simulink model "BEML_EMU"  (R2019b)
settings: configuration reference "ConfigSet_SimIntegration" (kept outside this file)
model workspace (MAT data in the model file):
  BrakesSampleTime = 0.01
  ConfigSampleTime = 0.05
  CouplingSampleTime = 0.05
  DoorsSampleTime = 0.05
  DynamicsSampleTime = 0.001
  ElectricalSampleTime = 0.05
  PRM_SimIntegration : Simulink.Parameter (value not decoded)
  PantographSampleTime = 0.05
  PneumaticsSampleTime = 0.01
  SampleTime = 0.001
  TractionSampleTime = 0.01
undefined symbols (not defined in the file): Acceleration, AngularAcceleration, AngularVelocity, BrakeFadeEnable, Brakes, BrakeShoeCoefficientCalculationMethod, BrakeShoeFrictionCoeff, BrakeTemperatureEnable, Common, DampingAdjustmentDesignMass, DavisCoeffA1, DavisCoeffA2, DavisCoeffB1, DavisCoeffB2, DavisCoefficients, DavisCoeffLeadCarC, DavisCoeffTailCarC, DiscIntNeverNeededParam, Doors, DragCalculationMethod, Dynamics, Effects, Electrical, EnableDampingAdjustmentByMass, Environment, Equipment, ExternalEffects, H, HasMotor, HasPanto, HornActivation, IsFirstVehicle, IsLastVehicle, isLeft, IsNonCab, LateralJolt, Location, LongitudinalJolt, MaxVehicles, MotionBaseSafetyCutout, OrientationDCM, P, Pantograph, Pneumatics, PneumaticsPoweredPanto, R, Traction, Transform, Tuning, UnitConfig, Velocity, VerticalJolt, VerticalJoltDown, VigilanceIntervention
libraries: simulink x35, IOStateMachinesLib x26, TestBenchLib x6, LatchesLib x3, BEML_EMU_BrakesInput_Lib x1, BEML_EMU_CBTCInterface_Lib x1, BEML_EMU_Couplers_Lib x1, BEML_EMU_DoorsInput_Lib x1, BEML_EMU_DynamicsInput_Lib x1, BEML_EMU_ElectricalInput_Lib x1, BEML_EMU_PantographInput_Lib x1, BEML_EMU_PneumaticsInput_Lib x1
(part 5 of 6)

== system BEML_EMU/InputsInterface/VehicleConfigProcessing/VehicleConfigInterface/VehicleConfigInterface/AssignTraction ==
  In Bus Element : Inport  PortName=VehicleConfig  Element=Common.Class
  Data Type Conversion : DataTypeConversion
  Merge1 : Merge  Inputs=4
  Switch Case2 : SwitchCase  CaseConditions={[101], [102], [103]}
  VehicleEquipment : Subsystem  mask(Tram Vehicle Equipment){HasMotors=on}
      mask prompts: HasMotors "Has Motors?"
      mask DialogControl ParameterGroupVar Prompt: Equipment
  VehicleEquipment1 : Subsystem  mask(Tram Vehicle Equipment){HasMotors=off}
      mask prompts: HasMotors "Has Motors?"
      mask DialogControl ParameterGroupVar Prompt: Equipment
  VehicleEquipment2 : Subsystem  mask(Tram Vehicle Equipment){HasMotors=on}
      mask prompts: HasMotors "Has Motors?"
      mask DialogControl ParameterGroupVar Prompt: Equipment
  VehicleEquipment3 : Subsystem  mask(Tram Vehicle Equipment){HasMotors=off}
      mask prompts: HasMotors "Has Motors?"
      mask DialogControl ParameterGroupVar Prompt: Equipment
  TractionBus : Outport  VectorParamsAs1DForOutWhenUnconnected=off
  wires:
  VehicleEquipment/1(EquipmentBus) -> Merge1/1
  Switch Case2/2 -> VehicleEquipment1/Action
  Merge1/1 -> TractionBus/1
  Switch Case2/4 -> VehicleEquipment3/Action
  Data Type Conversion/1 -> Switch Case2/1  "VehicleClasEnum"
  Switch Case2/3 -> VehicleEquipment2/Action
  In Bus Element/1 -> Data Type Conversion/1
  Switch Case2/1 -> VehicleEquipment/Action
  VehicleEquipment3/1(EquipmentBus) -> Merge1/4
  VehicleEquipment1/1(EquipmentBus) -> Merge1/2
  VehicleEquipment2/1(EquipmentBus) -> Merge1/3

== system BEML_EMU/InputsInterface/VehicleConfigProcessing/VehicleConfigInterface/VehicleConfigInterface/Common ==
  Input : Inport
  Bus Assignment3 : BusAssignment  AssignedSignals=NumberOfAxles
  Constant1 : Constant  Value=4  OutDataTypeStr=Inherit: Inherit via back propagation
  Data Type Conversion3 : DataTypeConversion
  Common : Outport  VectorParamsAs1DForOutWhenUnconnected=off
  wires:
  Constant1/1 -> Data Type Conversion3/1
  Data Type Conversion3/1 -> Bus Assignment3/2
  Bus Assignment3/1 -> Common/1
  Input/1 -> Bus Assignment3/1

== system BEML_EMU/InputsInterface/VehicleConfigProcessing/VehicleConfigInterface/VehicleConfigInterface/Dynamics ==
  note: Davis coefficients reused from BJSNA
      |
      | Davis Equation
      | F (N) = A1*Mass + A2 + B1*Mass*Vel + B2*Vel + C*Vel^2
  Dynamics : Inport
  TrainInput : Inport  Port=2
  Bus Assignment : BusAssignment  AssignedSignals=InitialVelocity
  Bus Assignment1 : BusAssignment  AssignedSignals=DragCalculationMethod,EnableDampingAdjustmentByMass,DampingAdjustmentDesignMass,DavisCoefficients
  Bus Assignment2 : BusAssignment  AssignedSignals=DavisCoeffA1,DavisCoeffA2,DavisCoeffB1,DavisCoeffB2,DavisCoeffLeadCarC,DavisCoeffTailCarC
  Bus Selector1 : BusSelector  OutputSignals=Overrides.InitialVelocity
  Constant : Constant  Value=0  OutDataTypeStr=Bus: BD_TrainDynamics_Cfg_Vehicle_DavisCoefficients
  Constant1 : Constant  Value=12.38
  Constant12 : Constant  Value=20e3
  Constant2 : Constant  Value=0
  Constant5 : Constant  Value=0.044e-3
  Constant6 : Constant  Value=5.18*0.8
  Constant7 : Constant  Value=5.18*0.2/7
  Constant8 : Constant  OutDataTypeStr=boolean
  Constant9 : Constant  Value=8.34e-3
  UseDavisCoeff : Constant  Value=DragCalculationMethod.Davis
  DynamicsProcessed : Outport  VectorParamsAs1DForOutWhenUnconnected=off
  wires:
  Dynamics/1 -> Bus Assignment/1
  Bus Selector1/1 -> Bus Assignment/2  "<InitialVelocity>"
  TrainInput/1 -> Bus Selector1/1
  Bus Assignment2/1 -> Bus Assignment1/5
  Constant/1 -> Bus Assignment2/1
  Constant1/1 -> Bus Assignment2/5
  UseDavisCoeff/1 -> Bus Assignment1/2
  Constant9/1 -> Bus Assignment2/2
  Constant2/1 -> Bus Assignment2/3
  Constant5/1 -> Bus Assignment2/4
  Constant7/1 -> Bus Assignment2/7
  Constant8/1 -> Bus Assignment1/3
  Constant6/1 -> Bus Assignment2/6
  Constant12/1 -> Bus Assignment1/4
  Bus Assignment1/1 -> DynamicsProcessed/1
  Bus Assignment/1 -> Bus Assignment1/1

== system BEML_EMU/InputsInterface/VehicleConfigProcessing/VehicleConfigInterface/VehicleConfigInterface/LocationConfig ==
  VehicleEnabled : Inport
  VehicleEnabledUp : Inport  Port=2
  VehicleEnabledDown : Inport  Port=3
  ClassDown : Inport  Port=4
  ClassUp : Inport  Port=5
  UnitID : Inport  Port=6
  In Bus Element1 : Inport  Port=7  PortName=VehicleConfig  Element=Common
  MaxUnit : Inport  Port=8
  AND2 : Logic  AllPortsSameDT=off  OutDataTypeStr=boolean
  AND3 : Logic  AllPortsSameDT=off  OutDataTypeStr=boolean
  Bus Assignment : BusAssignment  AssignedSignals=IsFirstVehicle,IsLastVehicle
  Bus Assignment1 : BusAssignment  AssignedSignals=UnitConfig.UnitID,UnitConfig.UnitConnection
  Constant1 : Constant  Value=0  OutDataTypeStr=Bus: BD_SimIntegration_Cfg_Vehicle_Location
  NOT : Logic  Operator=NOT  AllPortsSameDT=off  OutDataTypeStr=boolean
  NOT1 : Logic  Operator=NOT  AllPortsSameDT=off  OutDataTypeStr=boolean
  Subsystem : Subsystem
  UnitConf : Subsystem
  LocationConfig : Outport  VectorParamsAs1DForOutWhenUnconnected=off
  Enabled : Outport  Port=2
  UnitConnection : Outport  Port=3
  wires:
  Bus Assignment/1 -> Bus Assignment1/1
  AND2/1 -> Bus Assignment/2  "IsFirstVehicle"
  AND3/1 -> Bus Assignment/3  "IsLastVehicle"
  VehicleEnabledDown/1 -> NOT1/1
  NOT/1 -> AND2/2
  VehicleEnabled/1 -> AND3/1, AND2/1
  Constant1/1 -> Bus Assignment/1
  VehicleEnabledUp/1 -> NOT/1
  NOT1/1 -> AND3/2
  UnitConf/1(UnitConnection) -> Bus Assignment1/3, UnitConnection/1  "UnitConnection"
  In Bus Element1/1 -> UnitConf/1(VehicleConfig)
  ClassDown/1 -> UnitConf/2(ClassDown)
  UnitConf/2(Enabled) -> Enabled/1
  ClassUp/1 -> UnitConf/3(ClassUp)
  Bus Assignment1/1 -> LocationConfig/1
  UnitID/1 -> Subsystem/1(UnitID)
  MaxUnit/1 -> Subsystem/2(MaxUnit)
  Subsystem/1(Out2) -> Bus Assignment1/2

== system BEML_EMU/InputsInterface/VehicleConfigProcessing/VehicleConfigInterface/VehicleEnabled/Subsystem ==
  VehicleConfig : Inport  Partition=on  PartitionDimension=1  PartitionWidth=1  PartitionOffset=0
  Bus Selector : BusSelector  OutputSignals=Common.Enabled
  For Each : ForEach  DisableCoverage=on
  Enabled : Outport  ConcatenationDimension=1  VectorParamsAs1DForOutWhenUnconnected=off
  wires:
  VehicleConfig/1 -> Bus Selector/1
  Bus Selector/1 -> Enabled/1  "<Enabled>"

== system BEML_EMU/InputsInterface/VehicleConfigProcessing/VehicleConfigInterface/VehicleEnabled/Subsystem1 ==
  VehicleConfig : Inport  Partition=on  PartitionDimension=1  PartitionWidth=1  PartitionOffset=0
  Bus Selector : BusSelector  OutputSignals=Common.Class
  For Each : ForEach  DisableCoverage=on
  Class : Outport  ConcatenationDimension=1  VectorParamsAs1DForOutWhenUnconnected=off
  wires:
  Bus Selector/1 -> Class/1  "<Class>"
  VehicleConfig/1 -> Bus Selector/1

== system BEML_EMU/SimulatorSystems/ScoringSystemInterface/TrainLevelScoring/For Each Subsystem/Subsystem ==
  <Bogie> : Inport
  Bus Selector1 : BusSelector  OutputSignals=Bogie
  Subsystem : Subsystem
  Out1 : Outport
  Out2 : Outport  Port=2
  wires:
  <Bogie>/1 -> Bus Selector1/1
  Bus Selector1/1 -> Subsystem/1(<Bogie>)  "<Bogie>"
  Subsystem/1(Out1) -> Out1/1
  Subsystem/2(Out2) -> Out2/1

== system BEML_EMU/SimulatorSystems/Subsystem/Input Adapter/MotionBaseInputAdapter/Effects In Processing ==
  note: external effects is "degraded track" and Rough track
  In Bus Element : Inport  PortName=MotionBaseInput  Element=Effects
  Bus Assignment4 : BusAssignment  AssignedSignals=ExternalEffects,LongitudinalJolt,LateralJolt,VerticalJolt,VerticalJoltDown
  Constant : Constant  Value=0  OutDataTypeStr=Bus: BD_MotionBase_In_Vehicle_Effects
  FIXME : TestBenchLib/FIXME
      settings: SourceProductName=Sydac Utilities
  Effects : Outport
  wires:
  Bus Assignment4/1 -> Effects/1  "Effects"
  Constant/1 -> Bus Assignment4/1
  In Bus Element/1 -> Bus Assignment4/2  "Effects"
  FIXME/1 -> Bus Assignment4/6, Bus Assignment4/5, Bus Assignment4/4, Bus Assignment4/3

== system BEML_EMU/SimulatorSystems/Subsystem/Input Adapter/MotionBaseInputAdapter/Environment Dynamics In Processing ==
  Bus Assignment4 : BusAssignment  AssignedSignals=Contact
  Constant10 : Constant  Value=0  OutDataTypeStr=Bus: BD_MotionBase_In_Vehicle_Environment
  Constant5 : Constant  Value=0
  Environment : Outport
  wires:
  Constant10/1 -> Bus Assignment4/1
  Constant5/1 -> Bus Assignment4/2  "Contact"
  Bus Assignment4/1 -> Environment/1  "Environment"

== system BEML_EMU/SimulatorSystems/Subsystem/Input Adapter/MotionBaseInputAdapter/Tuning In Processing ==
  In Bus Element : Inport  PortName=MotionBaseInput  Element=Tuning
  Bus Assignment4 : BusAssignment  AssignedSignals=HeadingRateLimit
  Constant5 : Constant  Value=0
  Environment : Outport
  wires:
  Bus Assignment4/1 -> Environment/1  "Environment"
  Constant5/1 -> Bus Assignment4/2  "Contact"
  In Bus Element/1 -> Bus Assignment4/1

== system BEML_EMU/SimulatorSystems/Subsystem/Input Adapter/MotionBaseInputAdapter/Vehicle Dynamics In Processing ==
  note: $dl = rd\theta$
      |
      | $\frac{1}{r}dl = d\theta$
      | $\int\frac{1}{r}dl = \int d\theta$
  In Bus Element4 : Inport  PortName=VehicleInput  Element=Dynamics.TrackData.Gradient
  In Bus Element3 : Inport  PortName=VehicleInput  Element=Dynamics.TrackData.Radius
  In Bus Element : Inport  Port=2  PortName=DynamicsInput  Element=Inertia.Velocity
  In Bus Element5 : Inport  Port=2  PortName=DynamicsInput  Element=Inertia.Velocity
  In Bus Element1 : Inport  Port=2  PortName=DynamicsInput  Element=Inertia.Acceleration
  In Bus Element2 : Inport  Port=2  PortName=DynamicsInput  Element=TrackGeometry.LateralAcceleration
  Bus Assignment1 : BusAssignment  AssignedSignals=Velocity,Acceleration,AngularVelocity,AngularAcceleration,Transform
  Constant2 : Constant  Value=[0, 0, 0]
  Constant3 : Constant  Value=[0, 0, 0]
  Constant7 : Constant  Value=0  OutDataTypeStr=Bus: BD_MotionBase_In_Vehicle_Dynamics
  Coordinate Transformations : Subsystem
  Discrete-Time Integrator : DiscreteIntegrator  SampleTime=-1  ICPrevOutput=DiscIntNeverNeededParam  ICPrevScaledInput=DiscIntNeverNeededParam
  Lateral Velocity : Constant  Value=0
  Mux : Mux  Inputs=3
  Mux1 : Mux  Inputs=3
  SafeDivide : MathOperationsLib/SafeDivide
      settings: SourceProductName=Math Operations
  Vertical Acceleration : Constant  Value=0
  Vertical Velocity : Constant  Value=0
  theta : Trigonometry  Operator=atan
  VehicleDynamics : Outport
  wires:
  Mux1/1 -> Bus Assignment1/3  "Acceleration"
  Coordinate Transformations/1(Transform) -> Bus Assignment1/6
  Discrete-Time Integrator/1 -> Coordinate Transformations/1(Heave)  "Heave"
  Mux/1 -> Bus Assignment1/2
  theta/1 -> Coordinate Transformations/2(Pitch)  "Pitch"
  SafeDivide/1 -> Discrete-Time Integrator/1
  Constant3/1 -> Bus Assignment1/5  "AngularAcceleration"
  Vertical Velocity/1 -> Mux/3  "Vertical Velocity"
  Vertical Acceleration/1 -> Mux1/3  "Vertical Acceleration"
  Constant7/1 -> Bus Assignment1/1
  Bus Assignment1/1 -> VehicleDynamics/1  "Vehicle"
  Constant2/1 -> Bus Assignment1/4  "AngularVelocity"
  Lateral Velocity/1 -> Mux/2  "Lateral Velocity"
  In Bus Element2/1 -> Mux1/2
  In Bus Element/1 -> Mux/1  "Longitudinal Velocity"
  In Bus Element1/1 -> Mux1/1  "Longitudinal Acceleration"
  In Bus Element5/1 -> SafeDivide/1
  In Bus Element3/1 -> SafeDivide/2
  In Bus Element4/1 -> theta/1

== system BEML_EMU/InputsInterface/VehicleConfigProcessing/VehicleConfigInterface/VehicleConfigInterface/AssignDoors/VehicleEquipment1 ==
  Action Port : ActionPort  ActionPortLabel=case [ 102 ]:
  Bus Assignment3 : BusAssignment  AssignedSignals=isLeft,NumberOfDoors
  Constant6 : Constant  Value=0  OutDataTypeStr=Bus: BD_DoorSystem_Cfg_Door
  Data Type Conversion2 : DataTypeConversion
  Data Type Conversion3 : DataTypeConversion
  HasCab : Constant  Value=IsLeft
  HasMotors : Constant  Value=NumberOfDoors
  EquipmentBus : Outport  VectorParamsAs1DForOutWhenUnconnected=off
  wires:
  HasMotors/1 -> Data Type Conversion2/1
  Constant6/1 -> Bus Assignment3/1
  Bus Assignment3/1 -> EquipmentBus/1
  HasCab/1 -> Data Type Conversion3/1
  Data Type Conversion3/1 -> Bus Assignment3/2
  Data Type Conversion2/1 -> Bus Assignment3/3

== system BEML_EMU/InputsInterface/VehicleConfigProcessing/VehicleConfigInterface/VehicleConfigInterface/AssignDoors/VehicleEquipment2 ==
  Action Port : ActionPort  ActionPortLabel=case [ 103 ]:
  Bus Assignment3 : BusAssignment  AssignedSignals=isLeft,NumberOfDoors
  Constant6 : Constant  Value=0  OutDataTypeStr=Bus: BD_DoorSystem_Cfg_Door
  Data Type Conversion2 : DataTypeConversion
  Data Type Conversion3 : DataTypeConversion
  HasCab : Constant  Value=IsLeft
  HasMotors : Constant  Value=NumberOfDoors
  EquipmentBus : Outport  VectorParamsAs1DForOutWhenUnconnected=off
  wires:
  Data Type Conversion2/1 -> Bus Assignment3/3
  Data Type Conversion3/1 -> Bus Assignment3/2
  HasCab/1 -> Data Type Conversion3/1
  Bus Assignment3/1 -> EquipmentBus/1
  Constant6/1 -> Bus Assignment3/1
  HasMotors/1 -> Data Type Conversion2/1

== system BEML_EMU/InputsInterface/VehicleConfigProcessing/VehicleConfigInterface/VehicleConfigInterface/AssignDoors/VehicleEquipment3 ==
  Action Port : ActionPort  ActionPortLabel=default:
  Bus Assignment3 : BusAssignment  AssignedSignals=isLeft,NumberOfDoors
  Constant6 : Constant  Value=0  OutDataTypeStr=Bus: BD_DoorSystem_Cfg_Door
  Data Type Conversion2 : DataTypeConversion
  Data Type Conversion3 : DataTypeConversion
  HasCab : Constant  Value=IsLeft
  HasMotors : Constant  Value=NumberOfDoors
  EquipmentBus : Outport  VectorParamsAs1DForOutWhenUnconnected=off
  wires:
  HasMotors/1 -> Data Type Conversion2/1
  Constant6/1 -> Bus Assignment3/1
  Bus Assignment3/1 -> EquipmentBus/1
  HasCab/1 -> Data Type Conversion3/1
  Data Type Conversion3/1 -> Bus Assignment3/2
  Data Type Conversion2/1 -> Bus Assignment3/3

== system BEML_EMU/InputsInterface/VehicleConfigProcessing/VehicleConfigInterface/VehicleConfigInterface/AssignDoors/VehicleEquipment4 ==
  Action Port : ActionPort  ActionPortLabel=case [ 101 ]:
  Bus Assignment3 : BusAssignment  AssignedSignals=isLeft,NumberOfDoors
  Constant6 : Constant  Value=0  OutDataTypeStr=Bus: BD_DoorSystem_Cfg_Door
  Data Type Conversion2 : DataTypeConversion
  Data Type Conversion3 : DataTypeConversion
  HasCab : Constant  Value=IsLeft
  HasMotors : Constant  Value=NumberOfDoors
  EquipmentBus : Outport  VectorParamsAs1DForOutWhenUnconnected=off
  wires:
  Data Type Conversion2/1 -> Bus Assignment3/3
  Data Type Conversion3/1 -> Bus Assignment3/2
  HasCab/1 -> Data Type Conversion3/1
  Bus Assignment3/1 -> EquipmentBus/1
  Constant6/1 -> Bus Assignment3/1
  HasMotors/1 -> Data Type Conversion2/1

== system BEML_EMU/InputsInterface/VehicleConfigProcessing/VehicleConfigInterface/VehicleConfigInterface/AssignElectrical/VehicleEquipment ==
  Index : Inport
  Action Port : ActionPort  ActionPortLabel=case [ 101 ]:
  Bus Assignment3 : BusAssignment  AssignedSignals=HasPanto,HasCab,IsNonCab,HasMotor,HasMainCompressor,HasPantoReservoir
  Constant6 : Constant  Value=0  OutDataTypeStr=Bus: BD_ElectricalSystem_Cfg_Vehicle
  Data Type Conversion{1..3,5,9} (5 alike) : DataTypeConversion
  HasCab : Constant  Value=HasCab
  HasMotors : Constant  Value=HasMotors
  HasPantoReservoir : Constant  Value=HasPantoReservoir
  HasPantograph : Constant  Value=HasPantograph
  HasSimpleCab : Constant  Value=HasMainCompressor
  If : If  IfExpression=u1<=1  ElseIfExpressions=u1<=5
  If Action Subsystem : Subsystem  TreatAsAtomicUnit=on
  If Action Subsystem1 : Subsystem  TreatAsAtomicUnit=on
  If Action Subsystem2 : Subsystem  TreatAsAtomicUnit=on
  Merge : Merge  Inputs=3
  NOT : Logic  Operator=NOT  IconShape=distinctive  AllPortsSameDT=off  OutDataTypeStr=boolean
  EquipmentBus : Outport  VectorParamsAs1DForOutWhenUnconnected=off
  wires:
  HasPantograph/1 -> Data Type Conversion5/1
  HasMotors/1 -> Data Type Conversion2/1
  HasSimpleCab/1 -> Data Type Conversion1/1
  Constant6/1 -> Bus Assignment3/1
  HasCab/1 -> Data Type Conversion3/1
  HasPantoReservoir/1 -> Data Type Conversion9/1
  Data Type Conversion3/1 -> NOT/1, Bus Assignment3/3
  Data Type Conversion5/1 -> Bus Assignment3/2
  Data Type Conversion2/1 -> Bus Assignment3/5
  Data Type Conversion9/1 -> Bus Assignment3/7
  Data Type Conversion1/1 -> Bus Assignment3/6
  NOT/1 -> Bus Assignment3/4
  Merge/1 -> EquipmentBus/1
  If Action Subsystem/1(Out1) -> Merge/1
  Index/1 -> If/1
  If/2 -> If Action Subsystem2/Action
  Bus Assignment3/1 -> If Action Subsystem1/1(In1), If Action Subsystem2/1(In1), If Action Subsystem/1(In1)
  If/1 -> If Action Subsystem/Action
  If Action Subsystem2/1(Out1) -> Merge/2
  If Action Subsystem1/1(Out1) -> Merge/3
  If/3 -> If Action Subsystem1/Action

== system BEML_EMU/InputsInterface/VehicleConfigProcessing/VehicleConfigInterface/VehicleConfigInterface/AssignElectrical/VehicleEquipment1 ==
  Index : Inport
  Action Port : ActionPort  ActionPortLabel=case [ 102 ]:
  Bus Assignment3 : BusAssignment  AssignedSignals=HasPanto,HasCab,IsNonCab,HasMotor,HasMainCompressor,HasPantoReservoir
  Constant6 : Constant  Value=0  OutDataTypeStr=Bus: BD_ElectricalSystem_Cfg_Vehicle
  Data Type Conversion{1..3,5,9} (5 alike) : DataTypeConversion
  HasCab : Constant  Value=HasCab
  HasMotors : Constant  Value=HasMotors
  HasPantoReservoir : Constant  Value=HasPantoReservoir
  HasPantograph : Constant  Value=HasPantograph
  HasSimpleCab : Constant  Value=HasMainCompressor
  If : If  IfExpression=u1<=2  ElseIfExpressions=u1<=4
  If Action Subsystem : Subsystem  TreatAsAtomicUnit=on
  If Action Subsystem1 : Subsystem  TreatAsAtomicUnit=on
  If Action Subsystem2 : Subsystem  TreatAsAtomicUnit=on
  Merge : Merge  Inputs=3
  NOT : Logic  Operator=NOT  IconShape=distinctive  AllPortsSameDT=off  OutDataTypeStr=boolean
  EquipmentBus : Outport  VectorParamsAs1DForOutWhenUnconnected=off
  wires:
  NOT/1 -> Bus Assignment3/4
  Data Type Conversion1/1 -> Bus Assignment3/6
  Data Type Conversion9/1 -> Bus Assignment3/7
  Data Type Conversion2/1 -> Bus Assignment3/5
  Data Type Conversion5/1 -> Bus Assignment3/2
  Data Type Conversion3/1 -> NOT/1, Bus Assignment3/3
  HasPantoReservoir/1 -> Data Type Conversion9/1
  HasCab/1 -> Data Type Conversion3/1
  Constant6/1 -> Bus Assignment3/1
  HasSimpleCab/1 -> Data Type Conversion1/1
  HasMotors/1 -> Data Type Conversion2/1
  HasPantograph/1 -> Data Type Conversion5/1
  Merge/1 -> EquipmentBus/1
  Bus Assignment3/1 -> If Action Subsystem/1(In1), If Action Subsystem2/1(In1), If Action Subsystem1/1(In1)
  Index/1 -> If/1
  If/1 -> If Action Subsystem/Action
  If Action Subsystem/1(Out1) -> Merge/1
  If Action Subsystem1/1(Out1) -> Merge/2
  If/2 -> If Action Subsystem1/Action
  If Action Subsystem2/1(Out1) -> Merge/3
  If/3 -> If Action Subsystem2/Action

== system BEML_EMU/InputsInterface/VehicleConfigProcessing/VehicleConfigInterface/VehicleConfigInterface/AssignElectrical/VehicleEquipment2 ==
  Action Port : ActionPort  ActionPortLabel=default:
  Bus Assignment3 : BusAssignment  AssignedSignals=HasPanto,HasCab,IsNonCab,HasMotor,HasMainCompressor,HasPantoReservoir
  Constant6 : Constant  Value=0  OutDataTypeStr=Bus: BD_ElectricalSystem_Cfg_Vehicle
  Data Type Conversion{1..3,5,9} (5 alike) : DataTypeConversion
  HasCab : Constant  Value=HasCab
  HasMotors : Constant  Value=HasMotors
  HasPantoReservoir : Constant  Value=HasPantoReservoir
  HasPantograph : Constant  Value=HasPantograph
  HasSimpleCab : Constant  Value=HasMainCompressor
  NOT : Logic  Operator=NOT  IconShape=distinctive  AllPortsSameDT=off  OutDataTypeStr=boolean
  EquipmentBus : Outport  VectorParamsAs1DForOutWhenUnconnected=off
  wires:
  NOT/1 -> Bus Assignment3/4
  Data Type Conversion1/1 -> Bus Assignment3/6
  Data Type Conversion9/1 -> Bus Assignment3/7
  Data Type Conversion2/1 -> Bus Assignment3/5
  Data Type Conversion5/1 -> Bus Assignment3/2
  Data Type Conversion3/1 -> NOT/1, Bus Assignment3/3
  HasPantoReservoir/1 -> Data Type Conversion9/1
  HasCab/1 -> Data Type Conversion3/1
  Bus Assignment3/1 -> EquipmentBus/1
  Constant6/1 -> Bus Assignment3/1
  HasSimpleCab/1 -> Data Type Conversion1/1
  HasMotors/1 -> Data Type Conversion2/1
  HasPantograph/1 -> Data Type Conversion5/1

== system BEML_EMU/InputsInterface/VehicleConfigProcessing/VehicleConfigInterface/VehicleConfigInterface/AssignElectrical/VehicleEquipment3 ==
  Index : Inport
  Action Port : ActionPort  ActionPortLabel=case [ 103 ]:
  Bus Assignment3 : BusAssignment  AssignedSignals=HasPanto,HasCab,IsNonCab,HasMotor,HasMainCompressor,HasPantoReservoir
  Constant6 : Constant  Value=0  OutDataTypeStr=Bus: BD_ElectricalSystem_Cfg_Vehicle
  Data Type Conversion{1..3,5,9} (5 alike) : DataTypeConversion
  HasCab : Constant  Value=HasCab
  HasMotors : Constant  Value=HasMotors
  HasPantoReservoir : Constant  Value=HasPantoReservoir
  HasPantograph : Constant  Value=HasPantograph
  HasSimpleCab : Constant  Value=HasMainCompressor
  If : If  IfExpression=u1<=2  ElseIfExpressions=u1<=4
  If Action Subsystem : Subsystem  TreatAsAtomicUnit=on
  If Action Subsystem1 : Subsystem  TreatAsAtomicUnit=on
  If Action Subsystem2 : Subsystem  TreatAsAtomicUnit=on
  Merge : Merge  Inputs=3
  NOT : Logic  Operator=NOT  IconShape=distinctive  AllPortsSameDT=off  OutDataTypeStr=boolean
  EquipmentBus : Outport  VectorParamsAs1DForOutWhenUnconnected=off
  wires:
  HasPantograph/1 -> Data Type Conversion5/1
  HasMotors/1 -> Data Type Conversion2/1
  HasSimpleCab/1 -> Data Type Conversion1/1
  Constant6/1 -> Bus Assignment3/1
  HasCab/1 -> Data Type Conversion3/1
  HasPantoReservoir/1 -> Data Type Conversion9/1
  Data Type Conversion3/1 -> NOT/1, Bus Assignment3/3
  Data Type Conversion5/1 -> Bus Assignment3/2
  Data Type Conversion2/1 -> Bus Assignment3/5
  Data Type Conversion9/1 -> Bus Assignment3/7
  Data Type Conversion1/1 -> Bus Assignment3/6
  NOT/1 -> Bus Assignment3/4
  If Action Subsystem2/1(Out1) -> Merge/3
  If/1 -> If Action Subsystem/Action
  If/2 -> If Action Subsystem1/Action
  If/3 -> If Action Subsystem2/Action
  If Action Subsystem1/1(Out1) -> Merge/2
  Index/1 -> If/1
  If Action Subsystem/1(Out1) -> Merge/1
  Bus Assignment3/1 -> If Action Subsystem/1(In1), If Action Subsystem2/1(In1), If Action Subsystem1/1(In1)
  Merge/1 -> EquipmentBus/1

== system BEML_EMU/InputsInterface/VehicleConfigProcessing/VehicleConfigInterface/VehicleConfigInterface/AssignEquipment/VehicleEquipment ==
  Action Port : ActionPort  ActionPortLabel=case [ 101 ]:
  Bus Assignment3 : BusAssignment  AssignedSignals=HasCab,HasBogie,HasMotors,HasPneumaticPanto,HasElectricPanto,HasMainCompressor,HasMainReservoir,HasPantoReservoir,HasBrakeSystem,NumberOfDoors,NumberOfTractionBogies,NumberOfBrakingBogies
  Constant6 : Constant  Value=0  OutDataTypeStr=Bus: BD_SimIntegration_Cfg_Vehicle_Equipment
  Data Type Conversion{1..12} (12 alike) : DataTypeConversion
  HasCab : Constant  Value=HasCab
  HasMotors : Constant  Value=HasBogie
  HasPantoReservoir : Constant  Value=HasMainReservoir
  HasPantoReservoir1 : Constant  Value=HasMainCompressor
  HasPantoReservoir2 : Constant  Value=HasPantoReservoir
  HasPantoReservoir3 : Constant  Value=NumberOfDoors
  HasPantoReservoir4 : Constant  Value=NumberOfTractionBogies
  HasPantograph : Constant  Value=HasPneumaticPanto
  HasPantograph1 : Constant  Value=HasElectricPanto
  HasSimpleCab : Constant  Value=HasBrakeSystem
  HasSimpleCab1 : Constant  Value=NumberOfBrakingBogies
  HasStaticInverter : Constant  Value=HasMotors
  EquipmentBus : Outport  VectorParamsAs1DForOutWhenUnconnected=off
  wires:
  HasPantograph/1 -> Data Type Conversion5/1
  HasMotors/1 -> Data Type Conversion2/1
  HasSimpleCab/1 -> Data Type Conversion1/1
  Constant6/1 -> Bus Assignment3/1
  Bus Assignment3/1 -> EquipmentBus/1
  HasCab/1 -> Data Type Conversion3/1
  HasStaticInverter/1 -> Data Type Conversion8/1
  HasPantoReservoir/1 -> Data Type Conversion9/1
  Data Type Conversion3/1 -> Bus Assignment3/2
  Data Type Conversion5/1 -> Bus Assignment3/5
  Data Type Conversion2/1 -> Bus Assignment3/3
  Data Type Conversion9/1 -> Bus Assignment3/8
  Data Type Conversion8/1 -> Bus Assignment3/4
  Data Type Conversion1/1 -> Bus Assignment3/10
  Data Type Conversion4/1 -> Bus Assignment3/6
  HasPantograph1/1 -> Data Type Conversion4/1
  Data Type Conversion6/1 -> Bus Assignment3/7
  HasPantoReservoir1/1 -> Data Type Conversion6/1
  HasPantoReservoir2/1 -> Data Type Conversion7/1
  Data Type Conversion7/1 -> Bus Assignment3/9
  HasPantoReservoir4/1 -> Data Type Conversion11/1
  HasPantoReservoir3/1 -> Data Type Conversion12/1
  HasSimpleCab1/1 -> Data Type Conversion10/1
  Data Type Conversion11/1 -> Bus Assignment3/12
  Data Type Conversion10/1 -> Bus Assignment3/13
  Data Type Conversion12/1 -> Bus Assignment3/11

== system BEML_EMU/InputsInterface/VehicleConfigProcessing/VehicleConfigInterface/VehicleConfigInterface/AssignEquipment/VehicleEquipment1 ==
  Action Port : ActionPort  ActionPortLabel=case [ 102 ]:
  Bus Assignment3 : BusAssignment  AssignedSignals=HasCab,HasBogie,HasMotors,HasPneumaticPanto,HasElectricPanto,HasMainCompressor,HasMainReservoir,HasPantoReservoir,HasBrakeSystem,NumberOfDoors,NumberOfTractionBogies,NumberOfBrakingBogies
  Constant6 : Constant  Value=0  OutDataTypeStr=Bus: BD_SimIntegration_Cfg_Vehicle_Equipment
  Data Type Conversion{1..12} (12 alike) : DataTypeConversion
  HasCab : Constant  Value=HasCab
  HasMotors : Constant  Value=HasBogie
  HasPantoReservoir : Constant  Value=HasMainReservoir
  HasPantoReservoir1 : Constant  Value=HasMainCompressor
  HasPantoReservoir2 : Constant  Value=HasPantoReservoir
  HasPantoReservoir3 : Constant  Value=NumberOfDoors
  HasPantoReservoir4 : Constant  Value=NumberOfTractionBogies
  HasPantograph : Constant  Value=HasPneumaticPanto
  HasPantograph1 : Constant  Value=HasElectricPanto
  HasSimpleCab : Constant  Value=HasBrakeSystem
  HasSimpleCab1 : Constant  Value=NumberOfBrakingBogies
  HasStaticInverter : Constant  Value=HasMotors
  EquipmentBus : Outport  VectorParamsAs1DForOutWhenUnconnected=off
  wires:
  Data Type Conversion12/1 -> Bus Assignment3/11
  Data Type Conversion10/1 -> Bus Assignment3/13
  Data Type Conversion11/1 -> Bus Assignment3/12
  HasSimpleCab1/1 -> Data Type Conversion10/1
  HasPantoReservoir3/1 -> Data Type Conversion12/1
  HasPantoReservoir4/1 -> Data Type Conversion11/1
  Data Type Conversion7/1 -> Bus Assignment3/9
  HasPantoReservoir2/1 -> Data Type Conversion7/1
  HasPantoReservoir1/1 -> Data Type Conversion6/1
  Data Type Conversion6/1 -> Bus Assignment3/7
  HasPantograph1/1 -> Data Type Conversion4/1
  Data Type Conversion4/1 -> Bus Assignment3/6
  Data Type Conversion1/1 -> Bus Assignment3/10
  Data Type Conversion8/1 -> Bus Assignment3/4
  Data Type Conversion9/1 -> Bus Assignment3/8
  Data Type Conversion2/1 -> Bus Assignment3/3
  Data Type Conversion5/1 -> Bus Assignment3/5
  Data Type Conversion3/1 -> Bus Assignment3/2
  HasPantoReservoir/1 -> Data Type Conversion9/1
  HasStaticInverter/1 -> Data Type Conversion8/1
  HasCab/1 -> Data Type Conversion3/1
  Bus Assignment3/1 -> EquipmentBus/1
  Constant6/1 -> Bus Assignment3/1
  HasSimpleCab/1 -> Data Type Conversion1/1
  HasMotors/1 -> Data Type Conversion2/1
  HasPantograph/1 -> Data Type Conversion5/1

== system BEML_EMU/InputsInterface/VehicleConfigProcessing/VehicleConfigInterface/VehicleConfigInterface/AssignEquipment/VehicleEquipment2 ==
  Action Port : ActionPort  ActionPortLabel=case [ 103 ]:
  Bus Assignment3 : BusAssignment  AssignedSignals=HasCab,HasBogie,HasMotors,HasPneumaticPanto,HasElectricPanto,HasMainCompressor,HasMainReservoir,HasPantoReservoir,HasBrakeSystem,NumberOfDoors,NumberOfTractionBogies,NumberOfBrakingBogies
  Constant6 : Constant  Value=0  OutDataTypeStr=Bus: BD_SimIntegration_Cfg_Vehicle_Equipment
  Data Type Conversion{1..12} (12 alike) : DataTypeConversion
  HasCab : Constant  Value=HasCab
  HasMotors : Constant  Value=HasBogie
  HasPantoReservoir : Constant  Value=HasMainReservoir
  HasPantoReservoir1 : Constant  Value=HasMainCompressor
  HasPantoReservoir2 : Constant  Value=HasPantoReservoir
  HasPantoReservoir3 : Constant  Value=NumberOfDoors
  HasPantoReservoir4 : Constant  Value=NumberOfTractionBogies
  HasPantograph : Constant  Value=HasPneumaticPanto
  HasPantograph1 : Constant  Value=HasElectricPanto
  HasSimpleCab : Constant  Value=HasBrakeSystem
  HasSimpleCab1 : Constant  Value=NumberOfBrakingBogies
  HasStaticInverter : Constant  Value=HasMotors
  EquipmentBus : Outport  VectorParamsAs1DForOutWhenUnconnected=off
  wires:
  HasPantograph/1 -> Data Type Conversion5/1
  HasMotors/1 -> Data Type Conversion2/1
  HasSimpleCab/1 -> Data Type Conversion1/1
  Constant6/1 -> Bus Assignment3/1
  Bus Assignment3/1 -> EquipmentBus/1
  HasCab/1 -> Data Type Conversion3/1
  HasStaticInverter/1 -> Data Type Conversion8/1
  HasPantoReservoir/1 -> Data Type Conversion9/1
  Data Type Conversion3/1 -> Bus Assignment3/2
  Data Type Conversion5/1 -> Bus Assignment3/5
  Data Type Conversion2/1 -> Bus Assignment3/3
  Data Type Conversion9/1 -> Bus Assignment3/8
  Data Type Conversion8/1 -> Bus Assignment3/4
  Data Type Conversion1/1 -> Bus Assignment3/10
  Data Type Conversion4/1 -> Bus Assignment3/6
  HasPantograph1/1 -> Data Type Conversion4/1
  Data Type Conversion6/1 -> Bus Assignment3/7
  HasPantoReservoir1/1 -> Data Type Conversion6/1
  HasPantoReservoir2/1 -> Data Type Conversion7/1
  Data Type Conversion7/1 -> Bus Assignment3/9
  HasPantoReservoir4/1 -> Data Type Conversion11/1
  HasPantoReservoir3/1 -> Data Type Conversion12/1
  HasSimpleCab1/1 -> Data Type Conversion10/1
  Data Type Conversion11/1 -> Bus Assignment3/12
  Data Type Conversion10/1 -> Bus Assignment3/13
  Data Type Conversion12/1 -> Bus Assignment3/11

== system BEML_EMU/InputsInterface/VehicleConfigProcessing/VehicleConfigInterface/VehicleConfigInterface/AssignEquipment/VehicleEquipment3 ==
  Action Port : ActionPort  ActionPortLabel=default:
  Bus Assignment3 : BusAssignment  AssignedSignals=HasCab,HasBogie,HasMotors,HasPneumaticPanto,HasElectricPanto,HasMainCompressor,HasMainReservoir,HasPantoReservoir,HasBrakeSystem,NumberOfDoors,NumberOfTractionBogies,NumberOfBrakingBogies
  Constant6 : Constant  Value=0  OutDataTypeStr=Bus: BD_SimIntegration_Cfg_Vehicle_Equipment
  Data Type Conversion{1..12} (12 alike) : DataTypeConversion
  HasCab : Constant  Value=HasCab
  HasMotors : Constant  Value=HasBogie
  HasPantoReservoir : Constant  Value=HasMainReservoir
  HasPantoReservoir1 : Constant  Value=HasMainCompressor
  HasPantoReservoir2 : Constant  Value=HasPantoReservoir
  HasPantoReservoir3 : Constant  Value=NumberOfDoors
  HasPantoReservoir4 : Constant  Value=NumberOfTractionBogies
  HasPantograph : Constant  Value=HasPneumaticPanto
  HasPantograph1 : Constant  Value=HasElectricPanto
  HasSimpleCab : Constant  Value=HasBrakeSystem
  HasSimpleCab1 : Constant  Value=NumberOfBrakingBogies
  HasStaticInverter : Constant  Value=HasMotors
  EquipmentBus : Outport  VectorParamsAs1DForOutWhenUnconnected=off
  wires:
  Data Type Conversion12/1 -> Bus Assignment3/11
  Data Type Conversion10/1 -> Bus Assignment3/13
  Data Type Conversion11/1 -> Bus Assignment3/12
  HasSimpleCab1/1 -> Data Type Conversion10/1
  HasPantoReservoir3/1 -> Data Type Conversion12/1
  HasPantoReservoir4/1 -> Data Type Conversion11/1
  Data Type Conversion7/1 -> Bus Assignment3/9
  HasPantoReservoir2/1 -> Data Type Conversion7/1
  HasPantoReservoir1/1 -> Data Type Conversion6/1
  Data Type Conversion6/1 -> Bus Assignment3/7
  HasPantograph1/1 -> Data Type Conversion4/1
  Data Type Conversion4/1 -> Bus Assignment3/6
  Data Type Conversion1/1 -> Bus Assignment3/10
  Data Type Conversion8/1 -> Bus Assignment3/4
  Data Type Conversion9/1 -> Bus Assignment3/8
  Data Type Conversion2/1 -> Bus Assignment3/3
  Data Type Conversion5/1 -> Bus Assignment3/5
  Data Type Conversion3/1 -> Bus Assignment3/2
  HasPantoReservoir/1 -> Data Type Conversion9/1
  HasStaticInverter/1 -> Data Type Conversion8/1
  HasCab/1 -> Data Type Conversion3/1
  Bus Assignment3/1 -> EquipmentBus/1
  Constant6/1 -> Bus Assignment3/1
  HasSimpleCab/1 -> Data Type Conversion1/1
  HasMotors/1 -> Data Type Conversion2/1
  HasPantograph/1 -> Data Type Conversion5/1

== system BEML_EMU/InputsInterface/VehicleConfigProcessing/VehicleConfigInterface/VehicleConfigInterface/AssignPanto/VehicleEquipment ==
  Action Port : ActionPort  ActionPortLabel=case [ 101 ]:
  Bus Assignment3 : BusAssignment  AssignedSignals=HasPanto,PneumaticsPoweredPanto,ElectricPoweredPanto
  Constant6 : Constant  Value=0  OutDataTypeStr=Bus: BD_PantographSystem_Cfg_Vehicle
  Data Type Conversion2 : DataTypeConversion
  Data Type Conversion3 : DataTypeConversion
  Data Type Conversion5 : DataTypeConversion
  HasCab : Constant  Value=PenumaticsPoweredPanto
  HasMotors : Constant  Value=ElectricPoweredPanto
  HasPantograph : Constant  Value=HasPanto
  EquipmentBus : Outport  VectorParamsAs1DForOutWhenUnconnected=off
  wires:
  Constant6/1 -> Bus Assignment3/1
  Bus Assignment3/1 -> EquipmentBus/1
  HasCab/1 -> Data Type Conversion3/1
  HasPantograph/1 -> Data Type Conversion5/1
  HasMotors/1 -> Data Type Conversion2/1
  Data Type Conversion5/1 -> Bus Assignment3/2
  Data Type Conversion3/1 -> Bus Assignment3/3
  Data Type Conversion2/1 -> Bus Assignment3/4

== system BEML_EMU/InputsInterface/VehicleConfigProcessing/VehicleConfigInterface/VehicleConfigInterface/AssignPanto/VehicleEquipment1 ==
  Action Port : ActionPort  ActionPortLabel=case [ 102 ]:
  Bus Assignment3 : BusAssignment  AssignedSignals=HasPanto,PneumaticsPoweredPanto,ElectricPoweredPanto
  Constant6 : Constant  Value=0  OutDataTypeStr=Bus: BD_PantographSystem_Cfg_Vehicle
  Data Type Conversion2 : DataTypeConversion
  Data Type Conversion3 : DataTypeConversion
  Data Type Conversion5 : DataTypeConversion
  HasCab : Constant  Value=PenumaticsPoweredPanto
  HasMotors : Constant  Value=ElectricPoweredPanto
  HasPantograph : Constant  Value=HasPanto
  EquipmentBus : Outport  VectorParamsAs1DForOutWhenUnconnected=off
  wires:
  Data Type Conversion2/1 -> Bus Assignment3/4
  Data Type Conversion5/1 -> Bus Assignment3/2
  Data Type Conversion3/1 -> Bus Assignment3/3
  HasCab/1 -> Data Type Conversion3/1
  Bus Assignment3/1 -> EquipmentBus/1
  Constant6/1 -> Bus Assignment3/1
  HasMotors/1 -> Data Type Conversion2/1
  HasPantograph/1 -> Data Type Conversion5/1

== system BEML_EMU/InputsInterface/VehicleConfigProcessing/VehicleConfigInterface/VehicleConfigInterface/AssignPanto/VehicleEquipment2 ==
  Action Port : ActionPort  ActionPortLabel=default:
  Bus Assignment3 : BusAssignment  AssignedSignals=HasPanto,PneumaticsPoweredPanto,ElectricPoweredPanto
  Constant6 : Constant  Value=0  OutDataTypeStr=Bus: BD_PantographSystem_Cfg_Vehicle
  Data Type Conversion2 : DataTypeConversion
  Data Type Conversion3 : DataTypeConversion
  Data Type Conversion5 : DataTypeConversion
  HasCab : Constant  Value=PenumaticsPoweredPanto
  HasMotors : Constant  Value=ElectricPoweredPanto
  HasPantograph : Constant  Value=HasPanto
  EquipmentBus : Outport  VectorParamsAs1DForOutWhenUnconnected=off
  wires:
  Data Type Conversion2/1 -> Bus Assignment3/4
  Data Type Conversion5/1 -> Bus Assignment3/2
  Data Type Conversion3/1 -> Bus Assignment3/3
  HasCab/1 -> Data Type Conversion3/1
  Bus Assignment3/1 -> EquipmentBus/1
  Constant6/1 -> Bus Assignment3/1
  HasMotors/1 -> Data Type Conversion2/1
  HasPantograph/1 -> Data Type Conversion5/1

== system BEML_EMU/InputsInterface/VehicleConfigProcessing/VehicleConfigInterface/VehicleConfigInterface/AssignPanto/VehicleEquipment3 ==
  Action Port : ActionPort  ActionPortLabel=case [ 103 ]:
  Bus Assignment3 : BusAssignment  AssignedSignals=HasPanto,PneumaticsPoweredPanto,ElectricPoweredPanto
  Constant6 : Constant  Value=0  OutDataTypeStr=Bus: BD_PantographSystem_Cfg_Vehicle
  Data Type Conversion2 : DataTypeConversion
  Data Type Conversion3 : DataTypeConversion
  Data Type Conversion5 : DataTypeConversion
  HasCab : Constant  Value=PenumaticsPoweredPanto
  HasMotors : Constant  Value=ElectricPoweredPanto
  HasPantograph : Constant  Value=HasPanto
  EquipmentBus : Outport  VectorParamsAs1DForOutWhenUnconnected=off
  wires:
  HasPantograph/1 -> Data Type Conversion5/1
  HasMotors/1 -> Data Type Conversion2/1
  Constant6/1 -> Bus Assignment3/1
  Bus Assignment3/1 -> EquipmentBus/1
  HasCab/1 -> Data Type Conversion3/1
  Data Type Conversion3/1 -> Bus Assignment3/3
  Data Type Conversion5/1 -> Bus Assignment3/2
  Data Type Conversion2/1 -> Bus Assignment3/4

== system BEML_EMU/InputsInterface/VehicleConfigProcessing/VehicleConfigInterface/VehicleConfigInterface/AssignPneumatics/VehicleEquipment ==
  Action Port : ActionPort  ActionPortLabel=case [ 101 ]:
  Bus Assignment3 : BusAssignment  AssignedSignals=Equipment.HasDriverCab,Equipment.HasBogie,Equipment.HasCompressor,Equipment.HasMainReservoir,Equipment.HasBrakeSystem,Equipment.HasPantograph
  Constant6 : Constant  Value=0  OutDataTypeStr=Bus: BD_PneumaticsSystem_Cfg_Vehicle
  Data Type Conversion{1..3,5,8..9} (6 alike) : DataTypeConversion
  HasCab : Constant  Value=HasCab
  HasMotors : Constant  Value=HasBogie
  HasPantoReservoir : Constant  Value=HasMainReservoir
  HasPantograph : Constant  Value=HasPantograph
  HasSimpleCab : Constant  Value=HasBrakeSystem
  HasStaticInverter : Constant  Value=HasCompressor
  EquipmentBus : Outport  VectorParamsAs1DForOutWhenUnconnected=off
  wires:
  HasPantograph/1 -> Data Type Conversion5/1
  HasMotors/1 -> Data Type Conversion2/1
  HasSimpleCab/1 -> Data Type Conversion1/1
  Constant6/1 -> Bus Assignment3/1
  Bus Assignment3/1 -> EquipmentBus/1
  HasCab/1 -> Data Type Conversion3/1
  HasStaticInverter/1 -> Data Type Conversion8/1
  HasPantoReservoir/1 -> Data Type Conversion9/1
  Data Type Conversion3/1 -> Bus Assignment3/2
  Data Type Conversion5/1 -> Bus Assignment3/7
  Data Type Conversion2/1 -> Bus Assignment3/3
  Data Type Conversion9/1 -> Bus Assignment3/5
  Data Type Conversion8/1 -> Bus Assignment3/4
  Data Type Conversion1/1 -> Bus Assignment3/6

== system BEML_EMU/InputsInterface/VehicleConfigProcessing/VehicleConfigInterface/VehicleConfigInterface/AssignPneumatics/VehicleEquipment1 ==
  Action Port : ActionPort  ActionPortLabel=case [ 102 ]:
  Bus Assignment3 : BusAssignment  AssignedSignals=Equipment.HasDriverCab,Equipment.HasBogie,Equipment.HasCompressor,Equipment.HasMainReservoir,Equipment.HasBrakeSystem,Equipment.HasPantograph
  Constant6 : Constant  Value=0  OutDataTypeStr=Bus: BD_PneumaticsSystem_Cfg_Vehicle
  Data Type Conversion{1..3,5,8..9} (6 alike) : DataTypeConversion
  HasCab : Constant  Value=HasCab
  HasMotors : Constant  Value=HasBogie
  HasPantoReservoir : Constant  Value=HasMainReservoir
  HasPantograph : Constant  Value=HasPantograph
  HasSimpleCab : Constant  Value=HasBrakeSystem
  HasStaticInverter : Constant  Value=HasCompressor
  EquipmentBus : Outport  VectorParamsAs1DForOutWhenUnconnected=off
  wires:
  Data Type Conversion1/1 -> Bus Assignment3/6
  Data Type Conversion8/1 -> Bus Assignment3/4
  Data Type Conversion9/1 -> Bus Assignment3/5
  Data Type Conversion2/1 -> Bus Assignment3/3
  Data Type Conversion5/1 -> Bus Assignment3/7
  Data Type Conversion3/1 -> Bus Assignment3/2
  HasPantoReservoir/1 -> Data Type Conversion9/1
  HasStaticInverter/1 -> Data Type Conversion8/1
  HasCab/1 -> Data Type Conversion3/1
  Bus Assignment3/1 -> EquipmentBus/1
  Constant6/1 -> Bus Assignment3/1
  HasSimpleCab/1 -> Data Type Conversion1/1
  HasMotors/1 -> Data Type Conversion2/1
  HasPantograph/1 -> Data Type Conversion5/1

== system BEML_EMU/InputsInterface/VehicleConfigProcessing/VehicleConfigInterface/VehicleConfigInterface/AssignPneumatics/VehicleEquipment2 ==
  Action Port : ActionPort  ActionPortLabel=case [ 103 ]:
  Bus Assignment3 : BusAssignment  AssignedSignals=Equipment.HasDriverCab,Equipment.HasBogie,Equipment.HasCompressor,Equipment.HasMainReservoir,Equipment.HasBrakeSystem,Equipment.HasPantograph
  Constant6 : Constant  Value=0  OutDataTypeStr=Bus: BD_PneumaticsSystem_Cfg_Vehicle
  Data Type Conversion{1..3,5,8..9} (6 alike) : DataTypeConversion
  HasCab : Constant  Value=HasCab
  HasMotors : Constant  Value=HasBogie
  HasPantoReservoir : Constant  Value=HasMainReservoir
  HasPantograph : Constant  Value=HasPantograph
  HasSimpleCab : Constant  Value=HasBrakeSystem
  HasStaticInverter : Constant  Value=HasCompressor
  EquipmentBus : Outport  VectorParamsAs1DForOutWhenUnconnected=off
  wires:
  HasPantograph/1 -> Data Type Conversion5/1
  HasMotors/1 -> Data Type Conversion2/1
  HasSimpleCab/1 -> Data Type Conversion1/1
  Constant6/1 -> Bus Assignment3/1
  Bus Assignment3/1 -> EquipmentBus/1
  HasCab/1 -> Data Type Conversion3/1
  HasStaticInverter/1 -> Data Type Conversion8/1
  HasPantoReservoir/1 -> Data Type Conversion9/1
  Data Type Conversion3/1 -> Bus Assignment3/2
  Data Type Conversion5/1 -> Bus Assignment3/7
  Data Type Conversion2/1 -> Bus Assignment3/3
  Data Type Conversion9/1 -> Bus Assignment3/5
  Data Type Conversion8/1 -> Bus Assignment3/4
  Data Type Conversion1/1 -> Bus Assignment3/6

== system BEML_EMU/InputsInterface/VehicleConfigProcessing/VehicleConfigInterface/VehicleConfigInterface/AssignPneumatics/VehicleEquipment3 ==
  Action Port : ActionPort  ActionPortLabel=default:
  Bus Assignment3 : BusAssignment  AssignedSignals=Equipment.HasDriverCab,Equipment.HasBogie,Equipment.HasCompressor,Equipment.HasMainReservoir,Equipment.HasBrakeSystem,Equipment.HasPantograph
  Constant6 : Constant  Value=0  OutDataTypeStr=Bus: BD_PneumaticsSystem_Cfg_Vehicle
  Data Type Conversion{1..3,5,8..9} (6 alike) : DataTypeConversion
  HasCab : Constant  Value=HasCab
  HasMotors : Constant  Value=HasBogie
  HasPantoReservoir : Constant  Value=HasMainReservoir
  HasPantograph : Constant  Value=HasPantograph
  HasSimpleCab : Constant  Value=HasBrakeSystem
  HasStaticInverter : Constant  Value=HasCompressor
  EquipmentBus : Outport  VectorParamsAs1DForOutWhenUnconnected=off
  wires:
  Data Type Conversion1/1 -> Bus Assignment3/6
  Data Type Conversion8/1 -> Bus Assignment3/4
  Data Type Conversion9/1 -> Bus Assignment3/5
  Data Type Conversion2/1 -> Bus Assignment3/3
  Data Type Conversion5/1 -> Bus Assignment3/7
  Data Type Conversion3/1 -> Bus Assignment3/2
  HasPantoReservoir/1 -> Data Type Conversion9/1
  HasStaticInverter/1 -> Data Type Conversion8/1
  HasCab/1 -> Data Type Conversion3/1
  Bus Assignment3/1 -> EquipmentBus/1
  Constant6/1 -> Bus Assignment3/1
  HasSimpleCab/1 -> Data Type Conversion1/1
  HasMotors/1 -> Data Type Conversion2/1
  HasPantograph/1 -> Data Type Conversion5/1

== system BEML_EMU/InputsInterface/VehicleConfigProcessing/VehicleConfigInterface/VehicleConfigInterface/AssignTraction/VehicleEquipment ==
  Action Port : ActionPort  ActionPortLabel=case [ 101 ]:
  Bus Assignment3 : BusAssignment  AssignedSignals=HasMotors
  Constant6 : Constant  Value=0  OutDataTypeStr=Bus: BD_TractionSystem_Cfg_Vehicle
  Data Type Conversion5 : DataTypeConversion
  HasPantograph : Constant  Value=HasMotors
  EquipmentBus : Outport  VectorParamsAs1DForOutWhenUnconnected=off
  wires:
  Data Type Conversion5/1 -> Bus Assignment3/2
  Bus Assignment3/1 -> EquipmentBus/1
  Constant6/1 -> Bus Assignment3/1
  HasPantograph/1 -> Data Type Conversion5/1

== system BEML_EMU/InputsInterface/VehicleConfigProcessing/VehicleConfigInterface/VehicleConfigInterface/AssignTraction/VehicleEquipment1 ==
  Action Port : ActionPort  ActionPortLabel=case [ 102 ]:
  Bus Assignment3 : BusAssignment  AssignedSignals=HasMotors
  Constant6 : Constant  Value=0  OutDataTypeStr=Bus: BD_TractionSystem_Cfg_Vehicle
  Data Type Conversion5 : DataTypeConversion
  HasPantograph : Constant  Value=HasMotors
  EquipmentBus : Outport  VectorParamsAs1DForOutWhenUnconnected=off
  wires:
  HasPantograph/1 -> Data Type Conversion5/1
  Constant6/1 -> Bus Assignment3/1
  Bus Assignment3/1 -> EquipmentBus/1
  Data Type Conversion5/1 -> Bus Assignment3/2

== system BEML_EMU/InputsInterface/VehicleConfigProcessing/VehicleConfigInterface/VehicleConfigInterface/AssignTraction/VehicleEquipment2 ==
  Action Port : ActionPort  ActionPortLabel=case [ 103 ]:
  Bus Assignment3 : BusAssignment  AssignedSignals=HasMotors
  Constant6 : Constant  Value=0  OutDataTypeStr=Bus: BD_TractionSystem_Cfg_Vehicle
  Data Type Conversion5 : DataTypeConversion
  HasPantograph : Constant  Value=HasMotors
  EquipmentBus : Outport  VectorParamsAs1DForOutWhenUnconnected=off
  wires:
  Data Type Conversion5/1 -> Bus Assignment3/2
  Bus Assignment3/1 -> EquipmentBus/1
  Constant6/1 -> Bus Assignment3/1
  HasPantograph/1 -> Data Type Conversion5/1

== system BEML_EMU/InputsInterface/VehicleConfigProcessing/VehicleConfigInterface/VehicleConfigInterface/AssignTraction/VehicleEquipment3 ==
  Action Port : ActionPort  ActionPortLabel=default:
  Bus Assignment3 : BusAssignment  AssignedSignals=HasMotors
  Constant6 : Constant  Value=0  OutDataTypeStr=Bus: BD_TractionSystem_Cfg_Vehicle
  Data Type Conversion5 : DataTypeConversion
  HasPantograph : Constant  Value=HasMotors
  EquipmentBus : Outport  VectorParamsAs1DForOutWhenUnconnected=off
  wires:
  HasPantograph/1 -> Data Type Conversion5/1
  Constant6/1 -> Bus Assignment3/1
  Bus Assignment3/1 -> EquipmentBus/1
  Data Type Conversion5/1 -> Bus Assignment3/2

== system BEML_EMU/InputsInterface/VehicleConfigProcessing/VehicleConfigInterface/VehicleConfigInterface/LocationConfig/Subsystem ==
  UnitID : Inport
  MaxUnit : Inport  Port=2
  Add : Sum
  Constant : Constant
  Constant1 : Constant  Value=2
  Logical Operator : Logic  AllPortsSameDT=off  OutDataTypeStr=boolean
  Relational Operator1 : RelationalOperator  Operator===  OutDataTypeStr=boolean  RndMeth=Simplest
  Relational Operator2 : RelationalOperator  Operator===  OutDataTypeStr=boolean  RndMeth=Simplest
  Switch : Switch  Criteria=u2 > Threshold
  Out2 : Outport
  wires:
  Constant/1 -> Add/1
  Relational Operator1/1 -> Logical Operator/1
  MaxUnit/1 -> Relational Operator1/1
  Switch/1 -> Out2/1
  UnitID/1 -> Relational Operator2/1, Switch/3, Add/2
  Add/1 -> Switch/1
  Constant1/1 -> Relational Operator2/2, Relational Operator1/2
  Logical Operator/1 -> Switch/2
  Relational Operator2/1 -> Logical Operator/2
